simulink model "teamproject"  (R2020b)
settings: Solver=VariableStepAuto  StartTime=0.0  StopTime=Tstop  FixedStep=1e-6  RelTol=1e-3
PreLoadFcn:
  | k;
InitFcn:
  | k;
values from neighbouring files (symbols this model uses):
  Bbig = Bmotor.*iBig.^2 + Bgear.*iBig.^2    [k.m]
  Bsmall = Bmotor.*iSmall.^2 + Bgear.*iSmall.^2    [k.m]
  CF = 1300    [k.m]
  iBig = 30    [k.m]
  iSmall = 20    [k.m]
  Jbig = Jmotor.*iBig.^2 + Jgear.*iBig.^2 + Jarm + Jload    [k.m]
  Jsmall = Jmotor.*iSmall.^2 + Jgear.*iSmall.^2 + Jarm1 + Jload1    [k.m]
  K = 0.4    [k.m]
  K1 = 3    [k.m]
  Kd = 0.9    [k.m]
  Kd1 = 1.2    [k.m]
  Ki = 1.5    [k.m]
  Ki1 = 2    [k.m]
  Km = 42.9e-3    (= 0.0429)    [k.m]
  Kp = 2.1    [k.m]
  Kp1 = 2    [k.m]
  Lw = 0.514e-3    (= 0.000514)    [k.m]
  Rw = 2.68    [k.m]
  thetaD = pi/4    (= 0.785398163397)    [k.m]
libraries: cstblocks x2, pid_lib x2
settings Model: Creator=28217  LastModifiedBy=28217

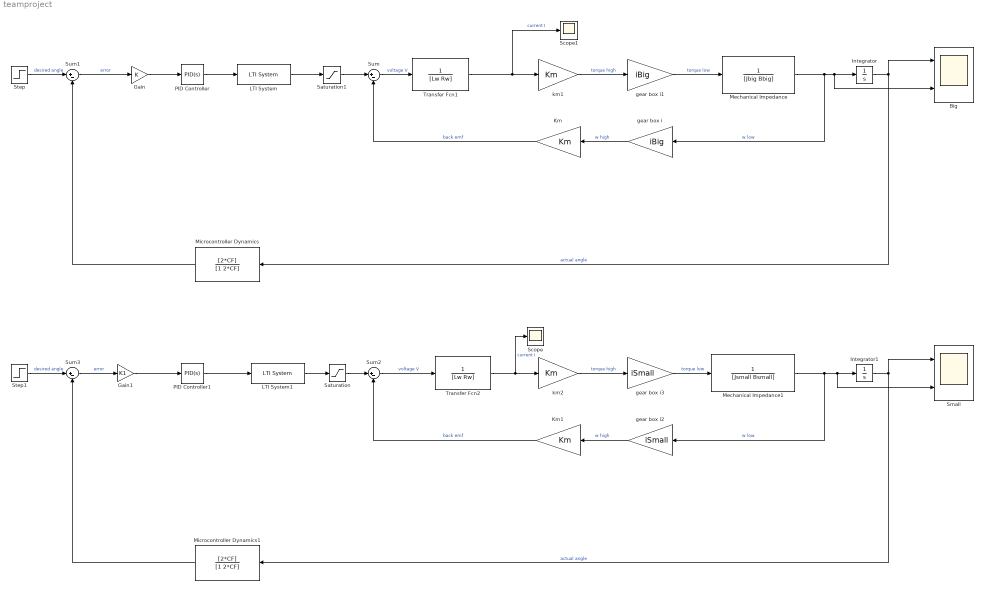
== system teamproject ==
  Big : Scope  NumInputPorts=2
  Gain : Gain  Gain=K
  Gain1 : Gain  Gain=K1
  Integrator : Integrator
  Integrator1 : Integrator
  Km : Gain  Gain=Km
  Km1 : Gain  Gain=Km
  LTI System : cstblocks/LTI System  sys=ampTF  IC=[]
  LTI System1 : cstblocks/LTI System  sys=ampTF  IC=[]
  Mechanical Impedance : TransferFcn  Denominator=[Jbig Bbig]
  Mechanical Impedance1 : TransferFcn  Denominator=[Jsmall Bsmall]
  Microcontroller Dynamics : TransferFcn  Numerator=[2*CF]  Denominator=[1 2*CF]
  Microcontroller Dynamics1 : TransferFcn  Numerator=[2*CF]  Denominator=[1 2*CF]
  PID Controller : pid_lib/PID Controller  Controller=PID  Form=Parallel  TimeDomain=Continuous-time  UseExternalTs=off  SampleTime=-1  IntegratorMethod=Forward Euler  FilterMethod=Forward Euler  ControllerParametersSource=internal  P=Kp  I=Ki  D=Kd  UseFilter=on  N=2*CF  TunerSelectOption=Frequency Response Based  InitialConditionSource=internal  InitialConditionForIntegrator=0  InitialConditionForFilter=0  DifferentiatorICPrevScaledInput=0  ExternalReset=none  TrackingMode=off  Kt=1  LimitOutput=off  SatLimitsSource=internal  UpperSaturationLimit=inf  LowerSaturationLimit=-inf  LinearizeAsGain=on  AntiWindupMode=none  Kb=1  POutMin=[]  POutMax=[]  IOutMin=[]  IOutMax=[]  DOutMin=[]  DOutMax=[]  NOutMin=[]  NOutMax=[]  SumOutMin=[]  SumOutMax=[]  SaturationOutMin=[]  SaturationOutMax=[]  PParamMin=[]  PParamMax=[]  IParamMin=[]  IParamMax=[]  DParamMin=[]  DParamMax=[]  NParamMin=[]  NParamMax=[]  KbParamMin=[]  KbParamMax=[]  KtParamMin=[]  KtParamMax=[]  KbOutMin=[]  KbOutMax=[]  KtOutMin=[]  KtOutMax=[]  IntegratorOutMin=[]  IntegratorOutMax=[]  FilterOutMin=[]  FilterOutMax=[]  SumI1OutMin=[]  SumI1OutMax=[]  SumI2OutMin=[]  SumI2OutMax=[]  SumI3OutMin=[]  SumI3OutMax=[]  SumI4OutMin=[]  SumI4OutMax=[]  SumDOutMin=[]  SumDOutMax=[]  DifferentiatorOutMin=[]  DifferentiatorOutMax=[]  FilterDiffOutCoefMin=[]  FilterDiffOutCoefMax=[]  ReciprocalOutMin=[]  ReciprocalOutMax=[]  SumDenOutMin=[]  SumDenOutMax=[]  SumNumOutMin=[]  SumNumOutMax=[]  DivideOutMin=[]  DivideOutMax=[]  UdiffTsProdOutMin=[]  UdiffTsProdOutMax=[]  NTsProdOutMin=[]  NTsProdOutMax=[]  UintegralTsProdOutMin=[]  UintegralTsProdOutMax=[]  UngainTsProdOutMin=[]  UngainTsProdOutMax=[]  IntegratorContinuousStateAttributes=''  IntegratorStateMustResolveToSignalObject=off  IntegratorRTWStateStorageClass=Auto  FilterContinuousStateAttributes=''  FilterStateMustResolveToSignalObject=off  FilterRTWStateStorageClass=Auto  ParallelPVariant=InternalParameters  IdealPVariant=Disabled  IVariant=InternalParameters  DVariant=InternalParameters  IntegratorVariant=Continuous  SatVariant=Disabled  AWVariant=Passthrough  PCopyVariant=Disabled  TRVariant=Disabled  FdbkBlocksVariant=Forward  IdealPFdbkVariant=Disabled  SatFdbkVariant=Disabled  DerivativeFilterVariant=ContFilter  NVariant=InternalParameters  NCopyVariant=Disabled  FilterICVariant=InternalICsFilter  IntegratorICVariant=InternalICs  ExternalResetVariant=Disabled  TRSumVariant=Passthrough  SumFdbkVariant=Disabled  SumVariant=Sum_PID  TsampFilterVariant=InternalTs  TsampNgainVariant=Passthrough  TsampIntegralVariant=Passthrough  ExternalSaturationOutDataTypeStr=Inherit: Same as second input
  PID Controller1 : pid_lib/PID Controller  Controller=PID  Form=Parallel  TimeDomain=Continuous-time  UseExternalTs=off  SampleTime=-1  IntegratorMethod=Forward Euler  FilterMethod=Forward Euler  ControllerParametersSource=internal  P=Kp1  I=Ki1  D=Kd1  UseFilter=on  N=2*CF  TunerSelectOption=Frequency Response Based  InitialConditionSource=internal  InitialConditionForIntegrator=0  InitialConditionForFilter=0  DifferentiatorICPrevScaledInput=0  ExternalReset=none  TrackingMode=off  Kt=1  LimitOutput=off  SatLimitsSource=internal  UpperSaturationLimit=inf  LowerSaturationLimit=-inf  LinearizeAsGain=on  AntiWindupMode=none  Kb=1  POutMin=[]  POutMax=[]  IOutMin=[]  IOutMax=[]  DOutMin=[]  DOutMax=[]  NOutMin=[]  NOutMax=[]  SumOutMin=[]  SumOutMax=[]  SaturationOutMin=[]  SaturationOutMax=[]  PParamMin=[]  PParamMax=[]  IParamMin=[]  IParamMax=[]  DParamMin=[]  DParamMax=[]  NParamMin=[]  NParamMax=[]  KbParamMin=[]  KbParamMax=[]  KtParamMin=[]  KtParamMax=[]  KbOutMin=[]  KbOutMax=[]  KtOutMin=[]  KtOutMax=[]  IntegratorOutMin=[]  IntegratorOutMax=[]  FilterOutMin=[]  FilterOutMax=[]  SumI1OutMin=[]  SumI1OutMax=[]  SumI2OutMin=[]  SumI2OutMax=[]  SumI3OutMin=[]  SumI3OutMax=[]  SumI4OutMin=[]  SumI4OutMax=[]  SumDOutMin=[]  SumDOutMax=[]  DifferentiatorOutMin=[]  DifferentiatorOutMax=[]  FilterDiffOutCoefMin=[]  FilterDiffOutCoefMax=[]  ReciprocalOutMin=[]  ReciprocalOutMax=[]  SumDenOutMin=[]  SumDenOutMax=[]  SumNumOutMin=[]  SumNumOutMax=[]  DivideOutMin=[]  DivideOutMax=[]  UdiffTsProdOutMin=[]  UdiffTsProdOutMax=[]  NTsProdOutMin=[]  NTsProdOutMax=[]  UintegralTsProdOutMin=[]  UintegralTsProdOutMax=[]  UngainTsProdOutMin=[]  UngainTsProdOutMax=[]  IntegratorContinuousStateAttributes=''  IntegratorStateMustResolveToSignalObject=off  IntegratorRTWStateStorageClass=Auto  FilterContinuousStateAttributes=''  FilterStateMustResolveToSignalObject=off  FilterRTWStateStorageClass=Auto  ParallelPVariant=InternalParameters  IdealPVariant=Disabled  IVariant=InternalParameters  DVariant=InternalParameters  IntegratorVariant=Continuous  SatVariant=Disabled  AWVariant=Passthrough  PCopyVariant=Disabled  TRVariant=Disabled  FdbkBlocksVariant=Forward  IdealPFdbkVariant=Disabled  SatFdbkVariant=Disabled  DerivativeFilterVariant=ContFilter  NVariant=InternalParameters  NCopyVariant=Disabled  FilterICVariant=InternalICsFilter  IntegratorICVariant=InternalICs  ExternalResetVariant=Disabled  TRSumVariant=Passthrough  SumFdbkVariant=Disabled  SumVariant=Sum_PID  TsampFilterVariant=InternalTs  TsampNgainVariant=Passthrough  TsampIntegralVariant=Passthrough  ExternalSaturationOutDataTypeStr=Inherit: Same as second input
  Saturation : Saturate  UpperLimit=40  LowerLimit=-40
  Saturation1 : Saturate  UpperLimit=40  LowerLimit=-40
  Scope : Scope
  Scope1 : Scope
  Small : Scope  NumInputPorts=2
  Step : Step  Time=0  After=thetaD  SampleTime=0
  Step1 : Step  Time=0  After=thetaD  SampleTime=0
  Sum{,1..3} (4 alike) : Sum  Inputs=|+-
  Transfer Fcn1 : TransferFcn  Denominator=[Lw Rw]
  Transfer Fcn2 : TransferFcn  Denominator=[Lw Rw]
  gear box i : Gain  Gain=iBig
  gear box i1 : Gain  Gain=iBig
  gear box i2 : Gain  Gain=iSmall
  gear box i3 : Gain  Gain=iSmall
  km1 : Gain  Gain=Km
  km2 : Gain  Gain=Km
  wires:
  Transfer Fcn1/1 -> Scope1/1, km1/1  "current I"
  km1/1 -> gear box i1/1  "torque high"
  gear box i1/1 -> Mechanical Impedance/1  "torque low"
  Sum/1 -> Transfer Fcn1/1  "voltage V"
  Km/1 -> Sum/2  "back emf"
  gear box i/1 -> Km/1  "w high"
  Mechanical Impedance/1 -> Big/2, Integrator/1, gear box i/1  "w low"
  PID Controller/1 -> LTI System/1
  Sum1/1 -> Gain/1  "error"
  Microcontroller Dynamics/1 -> Sum1/2
  Step/1 -> Sum1/1  "desired angle"
  Integrator/1 -> Big/1, Microcontroller Dynamics/1  "actual angle"
  Gain/1 -> PID Controller/1
  gear box i3/1 -> Mechanical Impedance1/1  "torque low"
  Gain1/1 -> PID Controller1/1
  Sum3/1 -> Gain1/1  "error"
  km2/1 -> gear box i3/1  "torque high"
  Mechanical Impedance1/1 -> Integrator1/1, Small/2, gear box i2/1  "w low"
  PID Controller1/1 -> LTI System1/1
  Microcontroller Dynamics1/1 -> Sum3/2
  Transfer Fcn2/1 -> Scope/1, km2/1  "current I"
  Km1/1 -> Sum2/2  "back emf"
  Sum2/1 -> Transfer Fcn2/1  "voltage V"
  Integrator1/1 -> Small/1, Microcontroller Dynamics1/1  "actual angle"
  Step1/1 -> Sum3/1  "desired angle"
  gear box i2/1 -> Km1/1  "w high"
  LTI System1/1 -> Saturation/1
  LTI System/1 -> Saturation1/1
  Saturation/1 -> Sum2/1
  Saturation1/1 -> Sum/1
